simulink model "simulation_mixed"  (Simulink 7.0)
settings: Solver=ode23s  StartTime=0.0  StopTime=400  RelTol=1e-3
libraries: cstblocks x2
settings Model: Creator=fromion  LastModifiedBy=vfromion  ExtModeTrigMode=oneshot  ExtModeArmWhenConnect=off  ExtModeAutoUpdateStatusClock=off
settings DataIOCC: LimitDataPoints=off
settings OptimizationCC: BlockReduction=off  BooleanDataType=off
settings DebuggingCC: SaveWithParameterizedLinksMsg=none  SignalResolutionControl=TryResolveAllWithWarning  SolverPrmCheckMsg=none  MultiTaskDSMMsg=warning  MultiTaskCondExecSysMsg=none
settings HardwareCC: TargetUnknown=on
settings RTWCC: IncludeERTFirstTime=on
settings GRTTargetCC: ModelReferenceCompliant=off  MatFileLogging=off

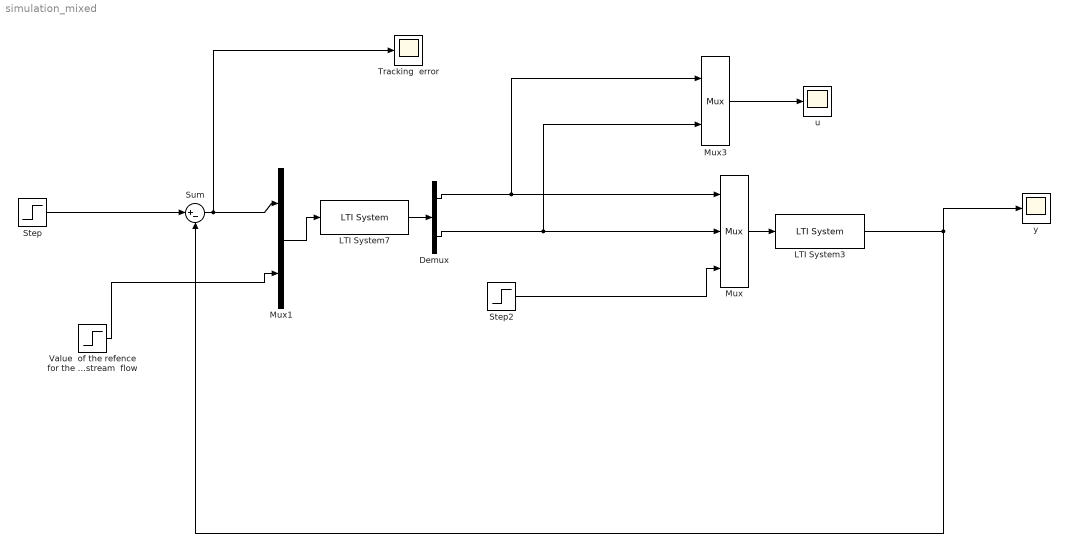
== system simulation_mixed ==
  Demux : Demux  Outputs=2
  LTI System3 : cstblocks/LTI System  SystemSampleTime=-1  sys=sys_synt_ss  IC=0
  LTI System7 : cstblocks/LTI System  SystemSampleTime=-1  sys=K_simul  IC=0
  Mux : Mux  Inputs=3
  Mux1 : Mux  Inputs=2
  Mux3 : Mux  Inputs=2
  Step : Step  SampleTime=0
  Step2 : Step  Time=100  SampleTime=0
  Sum : Sum  Inputs=|+-  SaturateOnIntegerOverflow=on  InputSameDT=on
  Tracking  error : Scope
      settings: TimeRange=400.8620689655172  YMin=-0.1985042735042735  YMax=1.192521367521368  SaveName=e  DataFormat=Array
  "Value  of the refence for the downstream  flow " : Step  Time=300  SampleTime=0
  u : Scope
      settings: TimeRange=400  YMin=-10  YMax=4  SaveName=y1  DataFormat=Array  SampleTime=0.1
  y : Scope
      settings: TimeRange=400  YMin=-0.2  YMax=1.2  SaveName=y  DataFormat=Array  SampleTime=0.1
  wires:
  Sum/1 -> Mux1/1, Tracking  error/1
  Step/1 -> Sum/1
  LTI System3/1 -> Sum/2, y/1
  Demux/2 -> Mux3/2, Mux/2
  "Value  of the refence for the downstream  flow "/1 -> Mux1/2
  Mux/1 -> LTI System3/1
  Demux/1 -> Mux/1, Mux3/1
  Mux1/1 -> LTI System7/1
  LTI System7/1 -> Demux/1
  Step2/1 -> Mux/3
  Mux3/1 -> u/1
